simulink model "TP4_control_kp"  (R2024b)
settings: Solver=VariableStepAuto  StartTime=0.0  StopTime=10.0  FixedStep=0.  RelTol=1e-3
undefined symbols (not defined in the file): states0, v0
settings Model: Creator=tomii  LastModifiedBy=tomii

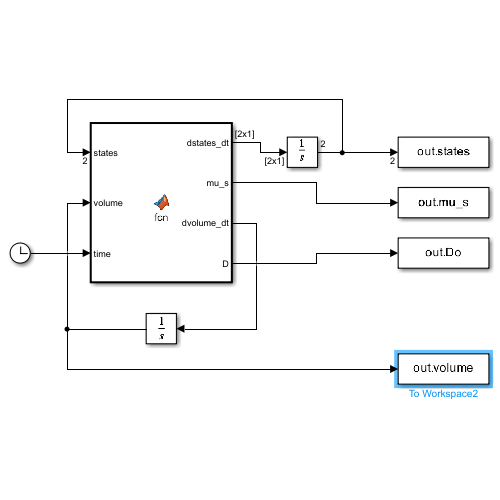
[thumbnail: Simulink's stored preview of the top-level diagram]
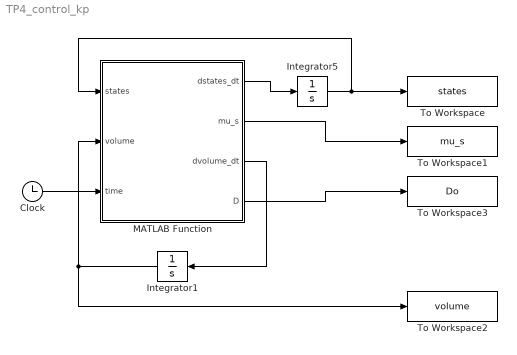
== system TP4_control_kp ==
  Clock : Clock
  Integrator1 : Integrator  InitialCondition=v0
  Integrator5 : Integrator  InitialCondition=states0
  MATLAB Function : MATLAB Function  TreatAsAtomicUnit=on
  To Workspace : ToWorkspace  VariableName=states  SaveFormat=Timeseries  SampleTime=-1
  To Workspace1 : ToWorkspace  VariableName=mu_s  SaveFormat=Timeseries  SampleTime=-1
  To Workspace2 : ToWorkspace  VariableName=volume  SaveFormat=Timeseries  SampleTime=-1
  To Workspace3 : ToWorkspace  VariableName=Do  SaveFormat=Timeseries  SampleTime=-1
  wires:
  MATLAB Function/1(dstates_dt) -> Integrator5/1
  Integrator5/1 -> MATLAB Function/1(states), To Workspace/1
  MATLAB Function/2(mu_s) -> To Workspace1/1
  MATLAB Function/4(D) -> To Workspace3/1
  Clock/1 -> MATLAB Function/3(time)
  MATLAB Function/3(dvolume_dt) -> Integrator1/1
  Integrator1/1 -> MATLAB Function/2(volume), To Workspace2/1

== matlab function TP4_control_kp/MATLAB Function ==
  data: dstates_dt output; mu_s output; dvolume_dt output; states input; volume input; time input; modelParameters parameter; D output
function [dstates_dt, mu_s, dvolume_dt, D] = fcn(states, volume, time, modelParameters)   
    
    K=modelParameters.K;
    xi_in=modelParameters.xi_in;
    ks1=modelParameters.ks1;

    kp=modelParameters.kp;

    mu_r=modelParameters.mu_r;
    s_r=modelParameters.s_r;
    x0=modelParameters.x0;
    v0=modelParameters.v0;
    s_in=modelParameters.s_in;

    Ks=modelParameters.mu_model.Ks;
    Kis=modelParameters.mu_model.Kis;
    mu_max=modelParameters.mu_model.mu_max;

    x=states(1);
    s=states(2);

    mu_s=mu_max*(s/(Ks+s+s*s/Kis));
    rx=x*mu_s;

    % X0=x0*v0;
    % D=(mu_r*X0*ks1*exp(mu_r*time))/((s_in-s_r)*volume)+(kp*(mu_r-mu_s))/((s_in-s_r));
    D = ks1*mu_r*x*(1+kp*(mu_r-mu_s))/(s_in-s_r);

    dstates_dt = K * rx + D*(xi_in-states);
    dvolume_dt = volume*D;

end
